simulink model "calibration"  (R2015b)
settings: Solver=ode1  StartTime=0.0  StopTime=Inf  FixedStep=0.001  RelTol=1e-3
PostLoadFcn:
  | , if any(exist('dsrtsu_mdlpostloadfcn', 'file') == [2, 3, 6]), try dsrtsu_mdlpostloadfcn('Execute', bdroot); catch fprintf('Error in PostLoadFcn (dsrtsu_mdlpostloadfcn) for model "%s":\n %s\n', bdroot, lasterr); end, end,
values from neighbouring files (symbols this model uses):
  BMS_CHARGING_TEMPERATURE_MAX_LIMIT = 50.0    (= 50)    [calibration_init.m]
  BMS_DISCHARGING_TEMPERATURE_MAX_LIMIT = 75.0    (= 75)    [calibration_init.m]
  BMS_MAX_OUTPUT_CURRENT_WARNING = 200.0    (= 200)    [calibration_init.m]
  BMS_SOH_MIN = 50.0    (= 50)    [calibration_init.m]
  BMS_STORED_ENERGY_MIN = 0.0    (= 0)    [calibration_init.m]
libraries: rtiflashlib x3
settings Model: DSRTSU_INTERNAL_RTI_VER=460  DSRTSU_INTERNAL_RTI_TYPE=rti1401  DSRTSU_INTERNAL_RTIFPGA=50  Creator=luis  LastModifiedBy=luis
settings DataIOCC: SaveOutput=off  SignalLogging=off  DSMLogging=off  SaveTime=off
settings OptimizationCC: BlockReduction=off  OptimizeBlockIOStorage=off  BufferReuse=off  GlobalBufferReuse=off  ExpressionFolding=off  LocalBlockOutputs=off
settings HardwareCC: ProdEndianess=BigEndian  ProdWordSize=32  ProdHWDeviceType=Generic->Custom  TargetIntDivRoundTo=Zero  TargetEndianess=BigEndian  TargetHWDeviceType=Generic->Custom
settings RTWCC: SystemTargetFile=rti1401.tlc  MakeCommand=make_rti  TemplateMakefile=rti1401.tmf  Description=dSPACE DS1401 Hardware Platform
settings STFCustomTargetCC: ParMdlRefBuildCompliant=on  ConcurrentExecutionCompliant=off  GeneratePreprocessorConditionals=Use local settings  MatFileLogging=on  CPPClassGenCompliant=off  SystemTargetFile=rti1401.tlc
settings GRTTargetCC: CompOptLevelCompliant=off  ConcurrentExecutionCompliant=off  CombineOutputUpdateFcns=off  CPPClassGenCompliant=off  GRTInterface=on  UseToolchainInfoCompliant=off  ExtModeMexFile=noextcomm

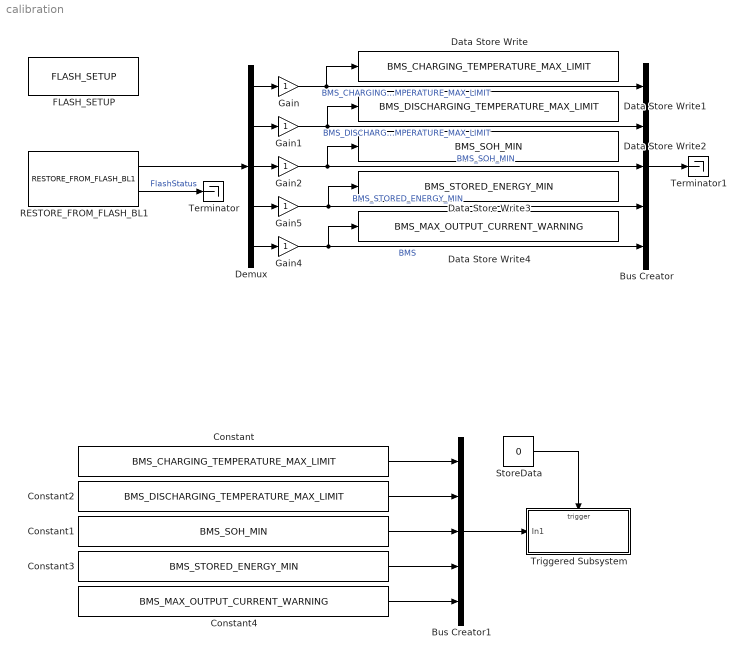
== system calibration ==
  Bus Creator : BusCreator  Inputs=5
  Bus Creator1 : BusCreator  Inputs=5
  Constant : Constant  Value=BMS_CHARGING_TEMPERATURE_MAX_LIMIT  SampleTime=-1
  Constant1 : Constant  Value=BMS_SOH_MIN  SampleTime=-1
  Constant2 : Constant  Value=BMS_DISCHARGING_TEMPERATURE_MAX_LIMIT  SampleTime=-1
  Constant3 : Constant  Value=BMS_STORED_ENERGY_MIN  SampleTime=-1
  Constant4 : Constant  Value=BMS_MAX_OUTPUT_CURRENT_WARNING  SampleTime=-1
  Data Store Write : DataStoreWrite  DataStoreName=BMS_CHARGING_TEMPERATURE_MAX_LIMIT
  Data Store Write1 : DataStoreWrite  DataStoreName=BMS_DISCHARGING_TEMPERATURE_MAX_LIMIT
  Data Store Write2 : DataStoreWrite  DataStoreName=BMS_SOH_MIN
  Data Store Write3 : DataStoreWrite  DataStoreName=BMS_STORED_ENERGY_MIN
  Data Store Write4 : DataStoreWrite  DataStoreName=BMS_MAX_OUTPUT_CURRENT_WARNING
  Demux : Demux  Outputs=5  BusSelectionMode=on
  FLASH_SETUP : rtiflashlib/FLASH_SETUP  UseNVRAM=on  UseFlrec=off  UseRestForFlRec=on  FlRecMemSize=1  BufferOverrunMode=Discard new data  TLCFileName=rtiflashsetup  Reserved1=[]  Reserved2=[]  Reserved3=[]  Reserved4=[]  DSProperties=struct('RTI',struct('Version',uint32(1),'BlockType',struct('isSLSource',uint8(0),'isSLSink',uint8(0),'isHWSource',uint8(0),'isHWSink',uint8(0),'isSetup',uint8(1),'isInline',uint8(1),'isNonInline',uint8(0),'isInterrupt',uint8(0),'isChannelwise',uint8(0)),'IOBoardType','DSFLASH','UnitType','FLASH','Identifier','SETUP','DialogType','SL','BlockSet','NONE','SlaveProcessor','NONE'))  RTIBlockInterface=struct('OutputPortsActive',0,'OutputPortsWidth',int32(0),'BlockDisplay',{{'Flash\nSetup','center'}},'IconTransparency','off','InitLevel',3,'BlockName',struct('Token',{{'FLASH_SETUP'}}),'MaskDescription',['Initializes the flash memory for flight recorder and non-volatile data interface blocks.'])  RTIBlockParameters=struct('UseNVRAM',{{logical(1),'ON',[0 1]}},'UseFlrec',{{logical(0),'ON',[0 1]}},'UseRestForFlRec',{{logical(1),'ON',[0 1]}},'FlRecMemSize',{{1,'OFF',[]}},'BufferOverrunMode',{{1,'OFF',[1 2]}},'TLCFileName',{{'rtiflashsetup','OFF',[]}})  RTISFcnParameters=struct('UseNVRAM','double','UseFlrec','double','UseRestForFlRec','double','FlRecMemSize','double','BufferOverrunMode','double','TLCFileName','char')  RTIBlockParaDefault=struct('UseNVRAM',0,'UseFlrec',1,'UseRestForFlRec',1,'FlRecMemSize',13,'BufferOverrunMode',1,'TLCFileName','rtiflashsetup')
  Gain{,1..2,4..5} (5 alike) : Gain
  RESTORE_FROM_FLASH_BL1 : rtiflashlib/RESTORE_FROM_FLASH_BL1  DataLabel=CAL_VALUES  NumOfElements=5  DataType=Double  DefaultValues="[ 0  0  0  0  0 ]"  TLCFileName=rtinvdatarestore  Reserved1=[]  Reserved2=[]  Reserved3=[]  Reserved4=[]  DSProperties=struct('RTI',struct('Version',uint32(1),'BlockType',struct('isSLSource',uint8(1),'isSLSink',uint8(0),'isHWSource',uint8(0),'isHWSink',uint8(0),'isSetup',uint8(0),'isInline',uint8(1),'isNonInline',uint8(0),'isInterrupt',uint8(0),'isChannelwise',uint8(0)),'IOBoardType','DSFLASH','UnitType','FLASH','Identifier','NVDATARESTORE','DialogType','SL','BlockSet','NONE','SlaveProcessor','NONE'))  RTIBlockInterface=struct('OutputPortsActive',[1 1],'OutputPortsWidth',int32([5 1]),'OutputPortsName',{{'CAL_VALUES','Status'}},'OutputPortsDataType',{{'SS_DOUBLE','SS_UINT16'}},'IconTransparency','on','InitLevel',3,'BlockName',struct('Token',{{'RESTORE_FROM_FLASH_BL1'}}),'MaskDescription',['To restore data from non-volatile flash memory'])  RTIBlockParameters=struct('DataLabel',{{'CAL_VALUES','OFF',[]}},'NumOfElements',{{5,'ON',[1 inf]}},'DataType',{{1,'OFF',[]}},'DefaultValues',{{[0 0 0 0 0],'OFF',[]}},'TLCFileName',{{'rtinvdatarestore','OFF',[]}})  RTISFcnParameters=struct('DataLabel','char','NumOfElements','double','DataType','double','DefaultValues','double','TLCFileName','char')  RTIBlockParaDefault=struct('DataLabel','Data','NumOfElements',1,'DataType',1,'DefaultValues',0,'TLCFileName','rtinvdatarestore')
  StoreData : Constant  Value=0
  Terminator : Terminator
  Terminator1 : Terminator
  Triggered Subsystem : Subsystem  TreatAsAtomicUnit=on
  wires:
  RESTORE_FROM_FLASH_BL1/1 -> Demux/1
  Demux/1 -> Gain/1
  Demux/2 -> Gain1/1
  Demux/3 -> Gain2/1
  Demux/4 -> Gain5/1
  Demux/5 -> Gain4/1
  Gain/1 -> Bus Creator/1, Data Store Write/1  "BMS_CHARGING_TEMPERATURE_MAX_LIMIT"
  Gain1/1 -> Data Store Write1/1, Bus Creator/2  "BMS_DISCHARGING_TEMPERATURE_MAX_LIMIT"
  Gain2/1 -> Data Store Write2/1, Bus Creator/3  "BMS_SOH_MIN"
  Gain5/1 -> Data Store Write3/1, Bus Creator/4  "BMS_STORED_ENERGY_MIN"
  Gain4/1 -> Data Store Write4/1, Bus Creator/5  "BMS"
  RESTORE_FROM_FLASH_BL1/2 -> Terminator/1  "FlashStatus"
  Bus Creator1/1 -> Triggered Subsystem/1(In1)
  Constant/1 -> Bus Creator1/1
  Constant2/1 -> Bus Creator1/2
  Constant1/1 -> Bus Creator1/3
  Constant3/1 -> Bus Creator1/4
  Constant4/1 -> Bus Creator1/5
  StoreData/1 -> Triggered Subsystem/Trigger
  Bus Creator/1 -> Terminator1/1

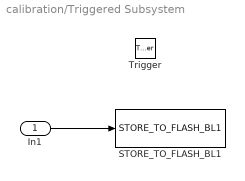
== system calibration/Triggered Subsystem ==
  In1 : Inport
  Trigger : TriggerPort
  STORE_TO_FLASH_BL1 : rtiflashlib/STORE_TO_FLASH_BL1  DataLabel=CAL_VALUES  NumOfElements=5  DataType=Double  TLCFileName=rtinvdatastore  Reserved1=[]  Reserved2=[]  Reserved3=[]  Reserved4=[]  DSProperties=struct('RTI',struct('Version',uint32(1),'BlockType',struct('isSLSource',uint8(0),'isSLSink',uint8(1),'isHWSource',uint8(0),'isHWSink',uint8(0),'isSetup',uint8(0),'isInline',uint8(1),'isNonInline',uint8(0),'isInterrupt',uint8(0),'isChannelwise',uint8(0)),'IOBoardType','DSFLASH','UnitType','FLASH','Identifier','NVDATASTORE','DialogType','SL','BlockSet','NONE','SlaveProcessor','NONE'))  RTIBlockInterface=struct('InputPortsActive',1,'InputPortsWidth',int32(5),'InputPortsName',{{'CAL_VALUES'}},'InputPortsDataType',{{'SS_DOUBLE'}},'IconTransparency','on','InitLevel',3,'BlockName',struct('Token',{{'STORE_TO_FLASH_BL1'}}),'MaskDescription',['To store data in non-volatile flash memory'])  RTIBlockParameters=struct('DataLabel',{{'CAL_VALUES','OFF',[]}},'NumOfElements',{{5,'ON',[1 inf]}},'DataType',{{1,'OFF',[]}},'TLCFileName',{{'rtinvdatastore','OFF',[]}})  RTISFcnParameters=struct('DataLabel','char','NumOfElements','double','DataType','double','TLCFileName','char')  RTIBlockParaDefault=struct('DataLabel','Data','NumOfElements',1,'DataType',1,'TLCFileName','rtinvdatastore')
  wires:
  In1/1 -> STORE_TO_FLASH_BL1/1
